simulink model "FFT4dSpace_1"  (R2021a)
settings: Solver=ode1  StartTime=0.0  StopTime=Inf  FixedStep=Ts  RelTol=1e-5
PostLoadFcn:
  | if any(exist('dsrtsu_mdlpostloadfcn', 'file') ~= 0), dsrtsu_mdlpostloadfcn('Execute', bdroot); end
InitFcn:
  | , if any(exist('rtifpga_mdlclblib', 'file') ~= 0), rtifpga_mdlclblib('Init', bdroot); end,
  | , if any(exist('dsmpb_private', 'file') ~= 0), dsmpb_private('dsmpb_mdlclblib', 'Init', bdroot); end,
values from neighbouring files (symbols this model uses):
  Ts_1kHz = 1e-3    (= 0.001)    [FFT4dSpace_1_i.m]
undefined symbols (not defined in the file or in its folder): CalibNormed, conv, mdlPara, PWMpara, Ro1_Be2, scaleHV, supplyPressure4VPPM
libraries: dsmpblib x46, tllib x2, dspxfrm3 x1, dspsigops x1
(part 1 of 2)
PreSaveFcn:
  | , if any(exist('dsmpb_private', 'file') ~= 0), dsmpb_private('dsmpb_mdlclblib', 'PreSave', bdroot); end,
CloseFcn:
  | , if any(exist('dsmpb_private', 'file') ~= 0), dsmpb_private('dsmpb_mdlclblib', 'Close', bdroot); end,
settings Model: TL_MAIN_DATA={'codeopt',{'globalbitfields',1,'cleancode',1},'logopt',{'globalloggingmode',4},'date',738813.6776019329,'advcodeopt',{'SupportSinglePrecisionLibraries';2}}  DS_PROJECTFILE=VEAE_Regler.dd  TLVersion=5.2.0.27  DSRTSU_INTERNAL_RTI_VER=580  DSRTSU_INTERNAL_RTI_TYPE=rti1202  RTICANMMDATA=struct('GeneralSetupData',struct('modelroot','C:\workspace\teachingSMC\FFT\dSpace\SCALEXIO','generalsettings',struct('filesettings',struct('destfolder',struct('Name','RTICANMM_FILES','Check',1),'buildfolder',struct('Name','.','Check',1),'AbsDestfolder',struct('Name','C:\workspace\teachingSMC\FFT\dSpace\SCALEXIO\RTICANMM_FILES'),'AbsBuildfolder',struct('Name','C:\workspace\teachingSMC\FFT\dSpace\SCALEXIO'))),'options',struct('addpaths',1,'rmpaths',1,'addtrcexclusion',true,'cannavigator',struct('checkmonitoring',0),'show_usrtrc',0,'use_usrtrc',0),'advanced',struct('options',ones(1,100)),'MPSetup',{{}},'RTI',struct('Type','DSRT','Ver','4.5','Date','02-May-2021'),'modelname','FFT4dSpace_1','block','FFT4dSpace_1'))  DSRTSU_INTERNAL_RTIFPGA=170  DSMPB_ID_DATA={'23691',struct('BlockId','e363dcf7-3c8b-40a0-94fa-9ca138f30a92','SignalIds',{{'8eaee084-b07d-4098-89ea-f14ffad18ffa'}}),'23692',struct('BlockId','33a1bf71-0d4c-4538-b9a6-2564a6bb3ed2','SignalIds',{{'7b532231-dc87-4623-a6bc-34b16234ae63'}}),'23693',struct('BlockId','80070c25-e06e-4fa7-bb77-63301d343f98','SignalIds',{{'1d35b1bf-c98b-4d88-ae94-1fc8c05d074d'}}),'23694',struct('BlockId','ad7704d0-4e59-4d7f-a1bb-c3e5207854ab','SignalIds',{{'30964f73-9c09-4fdc-bb51-0958be5a594d'}}),'23695',struct('BlockId','7aaee380-a7bb-4262-bf7a-0278c9ae6393','SignalIds',{{'cbf2b4e5-eba6-43e6-b587-c2127677f436'}}),'23696',struct('BlockId','36f2f2d5-5e42-4e25-9679-6cb3cb299ee5','SignalIds',{{'4b6b5e8b-c894-445c-bc7e-9990cb119b26'}}),'23697',struct('BlockId','71a2e424-6974-4253-bc43-95e389d7f603','SignalIds',{{'217da0a0-e3a9-4503-8c93-23feae479825'}}),'23698',struct('BlockId','8b7272b4-9be0-4b51-9ecb-302ecd5c3b3a','SignalIds',{{'4401bdaf-5b85-45f8-aa98-6959e1fe6847'}}),'23699',struct('BlockId','1db96408-7553-49ea-ae15-6e7e82f80655','SignalIds',{{'19da7aee-71cc-43f3-978b-66b6a099a4fa'}}),'23700',struct('BlockId','da4ac2f6-2b80-4d49-8dbf-3d2d4c3e429d','SignalIds',{{'0f867e66-a710-4dfd-aae0-36cd5f512122'}}),'23701',struct('BlockId','afd4257c-21a0-443f-8874-801e9e47d041','SignalIds',{{'ef4cd6d4-18a7-4dce-a9d8-4ae1aeb2dc70'}}),'23702',struct('BlockId','31438f08-e2ee-4bb4-abb9-b635e3636ed7','SignalIds',{{'7e1c8993-4ba1-482c-9dc1-fd8801ef3bb7'}}),'23722',struct('BlockId','bd682038-b3f1-451c-8889-2678fb1e0768','SignalIds',{{'8bc8299c-811b-4952-a633-8e6399a271bb','226ad07d-74a5-4348-9e16-0e760e13c5ea','fb77b335-58e6-40b8-9a39-c5d31b0115e1'}}),'23723',struct('BlockId','a9a2190b-8cc7-4831-ba2f-1a851ea58aef','SignalIds',{{'424d8948-39ab-4e70-baa5-0284423705d1','6157c886-271b-4e2c-9e64-a00fe997db60','bf2b604a-b232-4dca-951e-9f04b6190901'}}),'23724',struct('BlockId','4e0d0596-e847-41d4-ac4c-5549c7b68a70','SignalIds',{{'bcd34ae9-7391-4ec1-9116-0cf2ed083bb7','8dce8f9b-a3e1-43a5-9198-b0de8c72ab96','fd631e82-c4ba-420d-a832-f6f1a2e1fbf2'}}),'23725',struct('BlockId','b35cb07b-2765-4325-ba0e-4e1c0552a373','SignalIds',{{'bcc19acf-3645-4399-b2a6-a0b16bdb4434','a864334b-e486-47c0-b597-500b844d8df3','e9ee66d1-5c53-45d9-8a51-c60c45f2323a'}}),'23726',struct('BlockId','fc085d2d-a08d-447b-bb2c-55f41c3d2f58','SignalIds',{{'74f89104-11d1-44b2-9cce-5d5e36121983','58a323c5-8a29-4bfb-a24f-484cd4485a7a','a68058ee-dcad-46b1-af24-c0970f163968'}}),'23727',struct('BlockId','4f692a5d-2e07-4a4a-91aa-7aad3d22b323','SignalIds',{{'0b0ca5db-4351-48d9-aa89-15608aa96c34','c8c583e7-e575-4582-a023-d4cc5cccccc8','c457b778-0167-43a7-bc9f-1f9439149f83'}}),'23728',struct('BlockId','de7062cb-ec50-4fe6-ad2f-5964c9f43c03','SignalIds',{{'b0d0cdd9-a69b-4b2f-8686-152bd8c639ae','fd2f8604-b757-4c89-9a06-85e31da031f8','78e70a8d-34aa-48f6-9e91-9b7357999e14'}}),'23729',struct('BlockId','ee26962f-6483-47a5-9ae3-bdae23d41a82','SignalIds',{{'841699f9-1868-4e31-8b05-04831ea46d12','ef483acf-acac-49e3-bcf2-d459fa5b67e5','9a543403-5e94-4c76-83eb-20d980c5c198'}}),'23808',struct('BlockId','3618f7d3-770c-4d0b-a6f8-f57eef4aa707','SignalIds',{{'f887e2de-d35b-484c-8735-c498302bedaf'}}),'23809',struct('BlockId','d046d79b-4541-46bc-b50b-cbb132c517dd','SignalIds',{{'4adf8844-b3d9-48ac-afb0-aa431ebf3cfd'}}),'23810',struct('BlockId','9e33dab8-7c1e-4c10-8bac-9db27495f098','SignalIds',{{'c391cbb6-710b-41c5-a922-c0778a6fd7eb'}}),'23811',struct('BlockId','5047cf61-f79e-4571-babd-b46f8c31fe6f','SignalIds',{{'b6f989d1-85e3-4670-8a88-d8f123ece4d9'}}),'23812',struct('BlockId','84123028-2810-4ad1-975f-d307fc0b89eb','SignalIds',{{'9b0a0619-6ba6-4cbc-bb56-9b04bf7ffca0'}}),'23813',struct('BlockId','73b8bc57-ed34-4fde-ac01-a1e2ae6f212d','SignalIds',{{'f1bd759e-faf7-4478-8f9b-df97eda93df6'}}),'23814',struct('BlockId','02467e4c-1d3f-43c2-a575-9120e99575ea','SignalIds',{{'706fb417-39a5-419f-88e7-3d1a44326906'}}),'23815',struct('BlockId','30576d33-2aac-42bf-a78c-87ccc3cd6c01','SignalIds',{{'15c12989-3365-4ed1-9956-32a73db71a4d'}}),'23816',struct('BlockId','241ebb44-37d7-4bd2-a90d-0ea04f5a5d13','SignalIds',{{'f7f409fd-82fb-420b-ae76-eae684d90ce8'}}),'23817',struct('BlockId','fe42de6e-e6cd-4958-b6bb-718debe361a9','SignalIds',{{'2237635b-b2b4-4c94-86bb-2af412bd5cb8'}}),'23818',struct('BlockId','ea51ba60-b36a-4b1b-a248-4b35ae3fbf02','SignalIds',{{'80906cf2-aa07-496c-ab63-8acfe7b88759'}}),'23819',struct('BlockId','5e50a903-b4cf-479a-bba9-3e862b588a7a','SignalIds',{{'f80be48e-04e0-4bbc-94b1-e70b4d66f511'}}),'23820',struct('BlockId','7e573d54-38f9-41cf-a1ec-944dbb580650','SignalIds',{{'18737848-b3cc-470c-bff3-c14923aeca9b'}}),'23821',struct('BlockId','b40408dc-1d09-4b5e-b237-16e8872f357c','SignalIds',{{'381221ba-92f7-452a-8919-a8dd194524f7'}}),'23822',struct('BlockId','ac12e463-1157-45c4-a832-8a5484798087','SignalIds',{{'a20ec9ef-3c4b-4516-80e6-aea48d0d4a5c'}}),'23823',struct('BlockId','12f2115a-32be-4530-8d50-170bd71868ca','SignalIds',{{'394d649a-f46e-4805-83d9-d6cef483b7cd'}}),'23824',struct('BlockId','4e6ca114-81cb-481c-a0bb-b1573ff8e678','SignalIds',{{'da560366-0282-4fe5-94a0-da07a126ccc6'}}),'23825',struct('BlockId','6b18697c-40d5-402c-b9f7-e49b1f7cf619','SignalIds',{{'e3ede30a-e584-4b21-8fd4-4e675ebea708'}}),'23826',struct('BlockId','858f3f7c-a976-4e60-9a36-a5ba33175241','SignalIds',{{'e0824d91-0663-4ea2-af54-0f949cc3e418'}}),'23827',struct('BlockId','42c052ba-50d6-4985-9edf-50fac3901a3e','SignalIds',{{'2b1dcab9-ca84-4da1-a49d-55d11d9371e8'}}),'24118',struct('BlockId','47a249fb-d4e0-4e70-a5f5-36e301043995','SignalIds',{{'13cad4c5-6086-4e10-9ce6-5cdb82307704'}}),'24119',struct('BlockId','46dd8d37-e2a1-439f-89fc-ea00411d4ca3','SignalIds',{{'bbc1bd72-d794-442b-b6e2-735ad3ac33cb'}}),'24120',struct('BlockId','2aa52a3b-223d-4687-aa02-e1a44ea5c063','SignalIds',{{'bbf5d31c-0351-4836-994a-4c8856759900','550d0838-0baa-4757-a0e1-c46c9a3232a3'}}),'24121',struct('BlockId','995ad4dd-aaa8-465e-98cc-2dc6b2417123','SignalIds',{{'c825e840-241a-4b6f-bf2c-380bbaca74e6','5c01308f-615e-4599-acb8-22a35f81ada1'}}),'24122',struct('BlockId','885bc184-7968-4b50-898b-f403f006dcca','SignalIds',{{'6d9af1df-5ae3-49ad-ae84-01a7f8537bb7'}}),'25475',struct('BlockId','44a8e465-c9c5-409d-b2e8-7dd00d563f6d','SignalIds',{{'90fb2f1b-7fef-4790-ba3c-b5681fb51816','785fae22-0f32-4539-84e4-b96917a39273','b1ae88c2-cc42-4767-b4a8-823d65a01f97','176642e3-a060-49ad-bb31-43627c94ec8c','44d0cc4c-38bd-49d8-a6ec-c2148defedc4','7e07ee8a-8bd1-4ee4-aff1-5057cefc46ce'}})}  Creator=mibr  LastModifiedBy=nitr
settings SolverCC: AlgebraicLoopSolver=TrustRegion
settings DataIOCC: SaveFormat=Array  SaveOutput=off  DSMLogging=off  SaveTime=off  ReturnWorkspaceOutputs=off
settings OptimizationCC: BlockReduction=off  ConditionallyExecuteInputs=off  OptimizeBlockIOStorage=off  BufferReuse=off  GlobalBufferReuse=off  ExpressionFolding=off  LocalBlockOutputs=off  OptimizeDataStoreBuffers=off  BusAssignmentInplaceUpdate=off
settings DebuggingCC: SolverPrmCheckMsg=warning  TasksWithSamePriorityMsg=none  ParameterPrecisionLossMsg=none  UniqueDataStoreMsg=error  BusObjectLabelMismatch=error  StrictBusMsg=ErrorOnBusTreatedAsVector  NonBusSignalsTreatedAsBus=error  SFUnexpectedBacktrackingDiag=warning  SFNoUnconditionalDefaultTransitionDiag=warning  SFExecutionAtInitializationDiag=none  SFMachineParentedDataDiag=warning  ArithmeticOperatorsInVariantConditions=warning
settings HardwareCC: ProdBitPerPointer=32  ProdBitPerSizeT=32  ProdBitPerPtrDiffT=32  ProdLargestAtomicInteger=Integer  ProdWordSize=32  ProdLongLongMode=on  ProdHWDeviceType=Custom Processor->Custom  TargetIntDivRoundTo=Zero  TargetEndianess=BigEndian  TargetHWDeviceType=Custom Processor->Custom
settings ModelReferenceCC: EnableParallelModelReferenceBuilds=on
settings SFSimCC: MATLABDynamicMemAlloc=off  CustomCodeUndefinedFunction=UseInterfaceOnly
settings RTWCC: Description=dSPACE Run-Time Target (for VEOS on Windows and ConfigurationDesk)  SystemTargetFile=dsrt.tlc  GenCodeOnly=on  MakeCommand=make_dsrt  TemplateMakefile=dsrt_default_tmf  RTWVerbose=off
settings CodeAppCC: StateflowObjectComments=on
settings STFCustomTargetCC: ParMdlRefBuildCompliant=on  GRTInterface=off  UseToolchainInfoCompliant=off  SystemTargetFile=dsrt.tlc
settings GRTTargetCC: TargetLangStandard=C89/C90 (ANSI)  CompOptLevelCompliant=off  ConcurrentExecutionCompliant=off  CombineOutputUpdateFcns=off  MatFileLogging=off  CPPClassGenCompliant=off  UseToolchainInfoCompliant=off

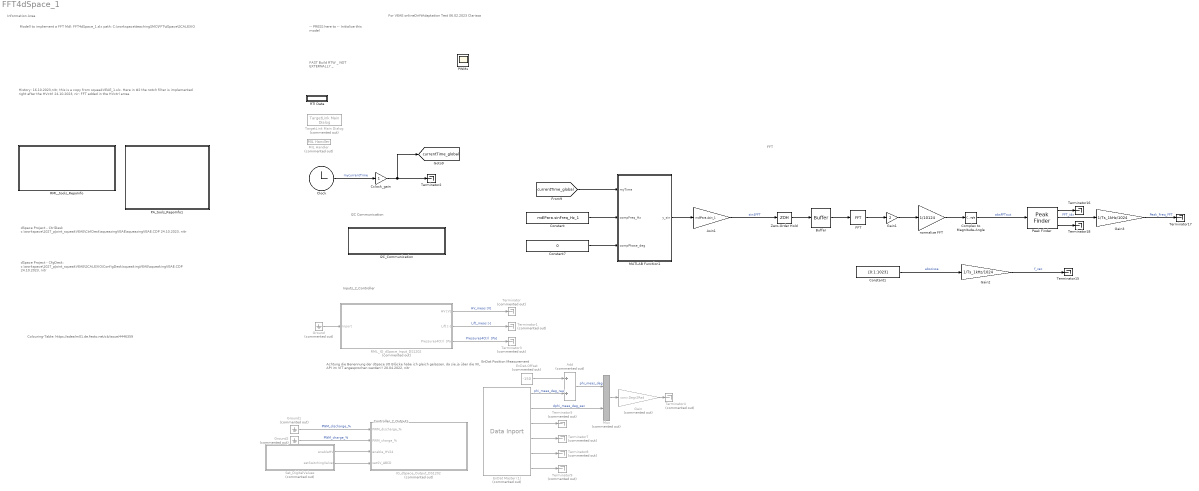
== system FFT4dSpace_1 ==
  note: Colouring-Table:
      | https://adealm01.de.festo.net/cb/issue/4446359
  note: EnDat Position Measurement
  note: For VEAE onlineDriftAdaptation Test
      | 06.02.2023
      |
      | Clarissa
  note: Achtung die Benennung der dSpace I/O Blöcke
      | habe ich gleich gelassen, da sie ja über die XIL API im VIT angesprochen werden!!
      |
      | 20.04.2022, nitr
  note: FAST Build RTW
      | _ NOT EXTERNALLY _
  note: Information Area
  note: dSpace Project - CtrlDesk
      | c:\workspace\1027_pJoint_squeakVEAE\CtrlDesk\squeazingVEAE\squeazingVEAE.CDP
      | 24.10.2023, nitr
  note: History:
      |
      | 16.10.2023,nitr, this is a copy from squeakVEAE_1.slx. Here in #2 the notch filter is implemented
      | right after the HVctrl
      | 24.10.2023, nir: FFT added in the HVctrl arrea
  note: Controller_2_Outputs
  note: -- PRESS here to --
      | Initialize this model
  note: Modell to implement a FFT
      |
      | Mdl: FFT4dSpace_1.slx
      | path: C:\workspace\teachingSMC\FFT\dSpace\SCALEXIO
  note: Inputs_2_Controller
  note: dSpace Project - CfgDesk:
      |
      | c:\workspace\1027_pJoint_squeakVEAE\SCALEXIO\ConfigDesk\squeakingVEAE\squeakingVEAE.CDP
      | 24.10.2023, nitr
  note: I2C Communication
  note: FFT
  Add : Sum  Commented=on
  Asin1 : Gain  Gain=mdlPara.Asin_1
  Buffer : Buffer  N=1024  OutputFrames=off
  Cclock_gain : Gain
  Clock : Clock
  Complex to Magnitude-Angle : ComplexToMagnitudeAngle  Output=Magnitude
  Constant : Constant  Value=mdlPara.sinFreq_Hz_1
  Constant1 : Constant  Value=[0:1:1023]
  Constant7 : Constant  Value=0
  EnDat Master (1) : dsmpblib/Data Inport  Priority=10000  Commented=on
      settings: SourceProductName=dSPACE Model Interface Blockset
  EnDat-Offset : Constant  Commented=on  Value=-150
  FFT : dspxfrm3/FFT  FFTImplementation=Auto  CompMethod=Table lookup  TableOpt=NEW  TableOptActive=Speed  BitRevOrder=off  Normalize=off  InheritFFTLength=on  FFTLength=64  WrapInput=on  roundingMode=Floor  overflowMode=off  firstCoeffDataTypeStr=Inherit: Same word length as input  firstCoeffLastDataTypeStr=Inherit: Same word length as input  outputMin=[]  outputMax=[]
  Gain : Gain  Commented=on  Gain=conv.Degr2Rad
  Gain1 : Gain  Gain=2
  Gain2 : Gain  Gain=1/Ts_1kHz/1024
  Gain3 : Gain  Gain=1/Ts_1kHz/1024
  Ground : Ground  Commented=on
  Ground1 : Ground  Commented=on
  Ground2 : Ground  Commented=on
  I2C_Communication : Subsystem
  IO_dSpace_Output_DS1202 : Subsystem  Tag=PA_IO_dSpace_Output_DS1513  Commented=on  mask(PA_dSpace_Output_DS1513){}
      mask help:
      | This block contains all outputsignals from dSpace RTI 1401. This Block
      | is a template. Before using in the block break the link to the library!
      | After breaking it is possible to connect the input with the block.
      |
      | It contains the signals:
      |
      | PWM_OUT1 ... PWM_OUT4
      | DIG_OUT1 ... DIG_OUT3
      | DAC1 ... DAC4
      mask Help: eval(['run(strcat(''',getenv('pasl_simulink'),''',''\documentation\tools\HelpForPaslElements.m''))']);
      mask Display: image('dSpaceInOut_rti1202_out.png')
  MATLAB Function1 : MATLAB Function  TreatAsAtomicUnit=on
  MIL Handler : tllib/MIL Handler  Commented=on  data={'date',738813.67760843749}
      settings: SourceProductName=dSPACE TargetLink common blockset
  Mux : Mux  Commented=on  Inputs=2
  PA_tools_RepoInfo1 : Subsystem  Tag=RevTagSubSys  mask(cover){}
      mask help: mask for library reasons
      settings: OpenFcn=PA_setRepoInfoBlock()
      mask Help: eval(['run(strcat(''',getenv('pasl_simulink'),''',''\documentation\tools\HelpForPaslElements.m''))']);
      mask Display: text(.05,.95,'Project:\n   Rev#:  8\n   RevID: 7424ff1b57da\n   date:  Mon, 23 Oct 2023 16:39:53 +0200\n   branch:  master\n\nPASL:\n   Rev#:  708\n   RevID: e154c95b446a\n   date:  Thu, 19 May 2022 11:39:18 +0200\n   branch:  master\n\nPATL:\n   Rev#:  144\n   RevID: 47544a47bed1\n   date:  Thu, 28 Apr 2022 22:19:34 +0200\n   branch:  master\n\nPADL:\n   Rev#:  UNKNOWN\n   RevID: UNKNOWN\n   date:  UNKNOWN\n   branch:  UNKNOWN\n\n','hor','left','ver','top')
  Peak Finder : dspsigops/Peak Finder  polarity=Maxima  indexBase=Zero  outputIdx=on  outputVal=on  maxPeaks=3  NoiseDistinguish=on  thresh=mdlPara.thres4peak  roundingMode=Floor  overflowMode=off
      settings: SourceProductBaseCode=DS  allowOverrides=off
  RML_IO_dSpace_Input_DS1202 : Subsystem  Commented=on
      mask Display: image('dSpaceInOut_rti1202_in.png')
  RML_tools_RepoInfo : Subsystem  Tag=rmlRevTagSubSys  mask(cover){}
      mask help: mask for library reasons
      settings: OpenFcn=rmlSetRepoInfoBlock()
      mask Help: eval(['run(strcat(''',getenv('rml_root'),'\documentation\tools\rmlHelpForRmlElements.m''))'])
      mask Display: text(.05,.95,'Project:\n   Rev#:  8\n   RevID: 7424ff1b57da\n   date:  Mon, 23 Oct 2023 16:39:53 +0200\n   branch:  master\n\nRML:\n   Rev#:  736\n   RevID: 95e677d319d7\n   date:  Fri, 24 Feb 2023 13:39:56 +0100\n   branch:  develop\n\n','hor','left','ver','top')
  RTI Data : Subsystem  Tag=struct('RTIDataServer',struct('RTIDataServerVs','2','RTIModelDescription','struct(''main'',''FFT4dSpace_1'',''sub'',''FFT4dSpace_1'',''isMp'',0)'))  LoadFcn="if exist('rtidc'), try,  rtidc('DataHostBlockClbLoad', gcbh); catch, disp(['Warning: ''LoadFcn'' for RTI Data block failed: ' lasterr]); end, end,"  mask(RTI_DATA_HOST){}
      mask help:
      | RTI Data Block.
      | This block is used by RTI to store internal model-dependent data.
      | Please keep this block on the root level of the model. Deleting this block will result in data loss.
      |
      | NEVER DELETE OR COPY THIS BLOCK!
      settings: CopyFcn="if exist('rtidc'), try,  rtidc('DataHostBlockClbCopy', gcbh); catch, disp(['Warning: ''CopyFcn'' for RTI Data block failed: ' lasterr]); end, end,"  DeleteFcn="if exist('rtidc'), try,  rtidc('DataHostBlockClbDelete', gcbh); catch, disp(['Warning: ''DeleteFcn'' for RTI Data block failed: ' lasterr]); end, end,"  ModelCloseFcn="if exist('rtidc'), try,  rtidc('DataHostBlockClbModelClose', gcbh); catch, disp(['Warning: ''ModelCloseFcn'' for RTI Data block failed: ' lasterr]); end, end,"  PreSaveFcn="if exist('rtidc'), try,  rtidc('DataHostBlockClbPreSave', gcbh); catch, disp(['Warning: ''PreSaveFcn'' for RTI Data block failed: ' lasterr]); end, end,"  PostSaveFcn="if exist('rtidc'), try,  rtidc('DataHostBlockClbPostSave', gcbh); catch, disp(['Warning: ''PostSaveFcn'' for RTI Data block failed: ' lasterr]); end, end,"  NameChangeFcn="if exist('rtidc'), try,  rtidc('DataHostBlockClbNameChange', gcbh); catch, disp(['Warning: ''NameChangeFcn'' for RTI Data block failed: ' lasterr]); end, end,"
      mask Help:
      | RTI Data Block.
      | This block is used by RTI to store internal model-dependent data.
      | Please keep this block on the root level of the model. Deleting this block will result in data loss.
      | 
      | NEVER DELETE OR COPY THIS BLOCK!
      mask Display:
      | text(0.5, 0.5, 'RTI Data', 'HorizontalAlignment', 'center');
      | plot([1 0]);
  Set_DigitalValues : Subsystem  Commented=on
  TargetLink Main Dialog : tllib/TargetLink Main Dialog  Commented=on  data=[]
      settings: SourceProductName=dSPACE TargetLink common blockset
  Terminator{,1,3..5,7..9} (8 alike) : Terminator  Commented=on
  Terminator{2,15..18} (5 alike) : Terminator
  Zero-Order Hold : ZeroOrderHold  SampleTime=Ts_1kHz
  normalize FFT : Gain  Gain=1/10124
  PWMs : Scope
  tag scope: currentTime_global=global
  wires:
  Ground2/1 -> IO_dSpace_Output_DS1202/2(PWM_charge_%)  "PWM_charge_%"
  RML_IO_dSpace_Input_DS1202/1(HV [V]) -> Terminator/1  "HV_meas [V]"
  RML_IO_dSpace_Input_DS1202/2(Lift [-]) -> Terminator1/1  "Lift_meas [-]"
  RML_IO_dSpace_Input_DS1202/3(Pressures4Ctrl  [Pa]) -> Terminator3/1  "Pressures4Ctrl  [Pa]"
  Ground1/1 -> IO_dSpace_Output_DS1202/1(PWM_discharge_%)  "PWM_discharge_%"
  Set_DigitalValues/1("enableHV ") -> IO_dSpace_Output_DS1202/3(enable_HV24)
  Set_DigitalValues/2(setSwitchingValves) -> IO_dSpace_Output_DS1202/4(setSV_ABCD)
  Clock/1 -> Cclock_gain/1  "mycurrentTime"
  Cclock_gain/1 -> [currentTime_global], Terminator2/1
  EnDat Master (1)/2 -> Mux/2  "dphi_meas_deg_sec"
  EnDat Master (1)/3 -> Terminator5/1
  EnDat Master (1)/4 -> Terminator7/1
  EnDat Master (1)/5 -> Terminator8/1
  EnDat Master (1)/6 -> Terminator9/1
  EnDat Master (1)/1 -> Add/2  "phi_meas_deg_raw"
  EnDat-Offset/1 -> Add/1
  Gain/1 -> Terminator4/1
  Mux/1 -> Gain/1
  Add/1 -> Mux/1  "phi_meas_deg"
  Ground/1 -> RML_IO_dSpace_Input_DS1202/1(Inport)
  Complex to Magnitude-Angle/1 -> Peak Finder/1  "absFFTout"
  Peak Finder/2 -> Gain3/1  "FFT_idx"
  Peak Finder/3 -> Terminator18/1
  FFT/1 -> Gain1/1
  normalize FFT/1 -> Complex to Magnitude-Angle/1
  Gain3/1 -> Terminator17/1  "Peak_Freq_FFT"
  Buffer/1 -> FFT/1
  Constant1/1 -> Gain2/1  "abscissa"
  Gain1/1 -> normalize FFT/1
  Gain2/1 -> Terminator15/1  "f_vec"
  Peak Finder/1 -> Terminator16/1
  Zero-Order Hold/1 -> Buffer/1
  Constant7/1 -> MATLAB Function1/3(compPhase_deg)
  Constant/1 -> MATLAB Function1/2(compFreq_Hz)
  [currentTime_global] -> MATLAB Function1/1(myTime)
  MATLAB Function1/1(y_sin) -> Asin1/1
  Asin1/1 -> Zero-Order Hold/1  "sin4FFT"

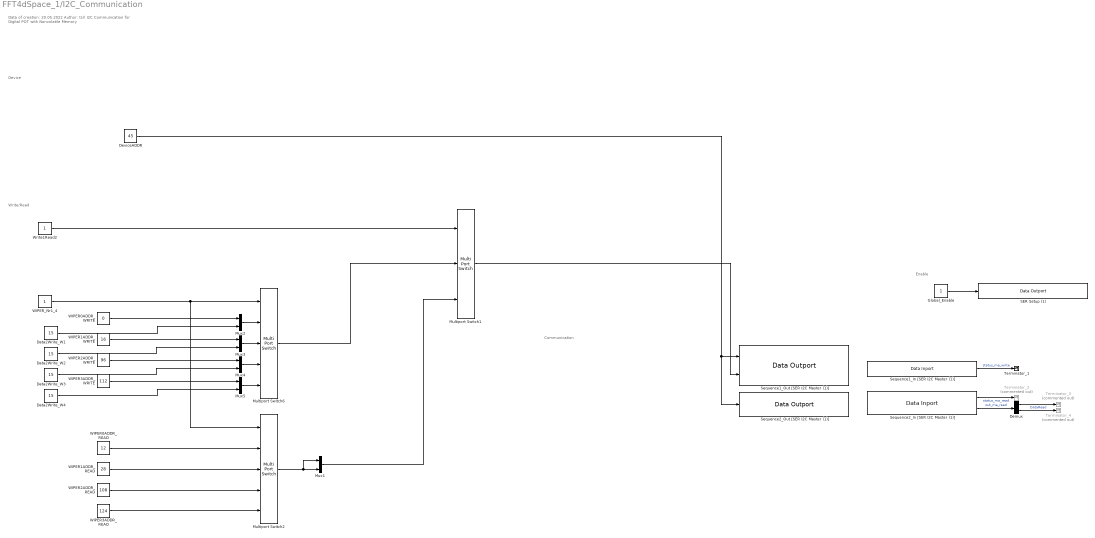
== system FFT4dSpace_1/I2C_Communication ==
  note: Data of creation: 20.05.2022
      | Author: tsrl
      |
      | I2C Communication for Digital POT with Nonvolatile Memory
  note: Enable
  note: Device
  note: Communication
  note: Write/Read
  Data2Write_W{1..4} (4 alike) : Constant  Value=15
  Demux : Demux  Outputs=2
  DeviceADDR : Constant  Value=45
  Global_Enable : Constant
  Multiport Switch1 : MultiPortSwitch  Inputs=2
  Multiport Switch2 : MultiPortSwitch  Inputs=4
  Multiport Switch6 : MultiPortSwitch  Inputs=4
  Mux{1..5} (5 alike) : Mux  Inputs=2
  SER Setup (1) : dsmpblib/Data Outport  Priority=-10000
      settings: SourceProductName=dSPACE Model Interface Blockset
  Sequence1_In [SER I2C Master (1)] : dsmpblib/Data Inport  Priority=10000
      settings: SourceProductName=dSPACE Model Interface Blockset
  Sequence1_Out [SER I2C Master (1)] : dsmpblib/Data Outport  Priority=-10000
      settings: SourceProductName=dSPACE Model Interface Blockset
  Sequence2_In [SER I2C Master (1)] : dsmpblib/Data Inport  Priority=10000
      settings: SourceProductName=dSPACE Model Interface Blockset
  Sequence2_Out [SER I2C Master (1)] : dsmpblib/Data Outport  Priority=-10000
      settings: SourceProductName=dSPACE Model Interface Blockset
  Terminator_1 : Terminator
  Terminator_2 : Terminator  Commented=on
  Terminator_3 : Terminator  Commented=on
  Terminator_4 : Terminator  Commented=on
  WIPER0ADDR_READ : Constant  Value=12
  WIPER0ADDR_WRITE : Constant  Value=0
  WIPER1ADDR_READ : Constant  Value=28
  WIPER1ADDR_WRITE : Constant  Value=16
  WIPER2ADDR_READ : Constant  Value=108
  WIPER2ADDR_WRITE : Constant  Value=96
  WIPER3ADDR_READ : Constant  Value=124
  WIPER3ADDR_WRITE : Constant  Value=112
  WIPER_Nr1_4 : Constant
  Write1Read2 : Constant
  wires:
  WIPER_Nr1_4/1 -> Multiport Switch2/1, Multiport Switch6/1
  Global_Enable/1 -> SER Setup (1)/1
  Sequence1_In [SER I2C Master (1)]/1 -> Terminator_1/1  "status_ma_write"
  WIPER3ADDR_READ/1 -> Multiport Switch2/5
  WIPER1ADDR_READ/1 -> Multiport Switch2/3
  Sequence2_In [SER I2C Master (1)]/1 -> Terminator_2/1  "status_ma_read"
  Multiport Switch2/1 -> Mux1/1, Mux1/2
  Mux1/1 -> Multiport Switch1/3
  WIPER2ADDR_READ/1 -> Multiport Switch2/4
  Write1Read2/1 -> Multiport Switch1/1
  WIPER0ADDR_READ/1 -> Multiport Switch2/2
  Demux/2 -> Terminator_4/1  "DataRead"
  DeviceADDR/1 -> Sequence2_Out [SER I2C Master (1)]/1, Sequence1_Out [SER I2C Master (1)]/1
  Multiport Switch1/1 -> Sequence1_Out [SER I2C Master (1)]/2
  Sequence2_In [SER I2C Master (1)]/2 -> Demux/1  "out_ma_read"
  Demux/1 -> Terminator_3/1
  Multiport Switch6/1 -> Multiport Switch1/2
  WIPER0ADDR_WRITE/1 -> Mux2/1
  Data2Write_W1/1 -> Mux2/2
  WIPER1ADDR_WRITE/1 -> Mux3/1
  WIPER2ADDR_WRITE/1 -> Mux4/1
  WIPER3ADDR_WRITE/1 -> Mux5/1
  Data2Write_W2/1 -> Mux3/2
  Data2Write_W3/1 -> Mux4/2
  Data2Write_W4/1 -> Mux5/2
  Mux2/1 -> Multiport Switch6/2
  Mux3/1 -> Multiport Switch6/3
  Mux4/1 -> Multiport Switch6/4
  Mux5/1 -> Multiport Switch6/5

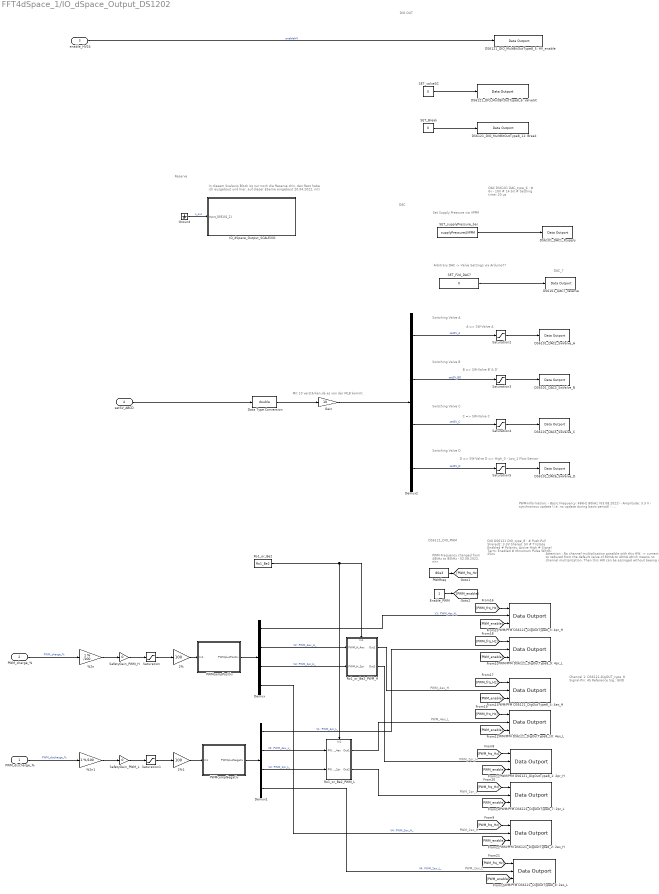
== system FFT4dSpace_1/IO_dSpace_Output_DS1202 ==
  note: A => SW-Valve A
  note: Reserve
  note: PWM Frequency changed from 48kHz to 80kHz - 02.08.2022, nitr
  note: In diesem Scalexio Block ist nur noch die Reserve drin,
      | den Rest habe ich ausgebaut und hier, auf dieser Eberne eingebaut
      | 20.04.2022, nitr
  note: Mit 10 verstärken,da es von der MLB kommt.
  note: Arbitrary DAC -> Valve Settings via Arduino??
  note: Set Supply Pressure via VPPM
  note: DAC
  note: DIG OUT
  note: PWM_4ex_H
  note: PWM_4ex_L
  note: PWM_2ex_H
  note: PWM_2pr_L
  note: PWM_2pr_H
  note: PWM_2ex_L
  note: DAC_7
  note: Switching Valve A
  note: Switching Valve B
  note: Switching Valve C
  note: Switching Valve D
  note: DAC DS6101 DAC_type_6 :
      | # 0v - 10V
      | # 14 bit
      | # Settling time: 20 µs
  note: DIO DS6121 DIO_type_8 :
      | # Push-Pull
      | Shared2: 3.3V
      | Shared: 5V
      | # Tristate Enabled
      | # Polarity: Active High
      | # Signal Term: Enabled
      |
      | # Minumum Pulse Witdh: 25ns
  note: Channel 1: DS6121-DigOUT_type_8
      | Signal-Pin: 45
      | Reference Sig.: GND
  note: PWM-Information:
      | - Basic Frequency: 48kHz 80kHz (03.08.2022)
      | - Amplitude: 3.3 V
      | - synchronous update (i.e. no update during basis period)
      | - ....
  note: DS6121_DIO_PWM
  note: Attention :
      | No channel multiplication possible with this HW,
      | -> current has to reduced from the default value of 80mA to 40mA
      | which means no channel multiplication. Then this HW can be assinged
      | without beeing red :)
  note: B => SW-Valve B' & D'
  note: C => SW-Valve C
  note: D => SW-Valve D => High_0 - Low_1 Flow Sensor
  PWM_discharge_% : Inport
  PWM_charge_% : Inport  Port=2
  enable_HV24 : Inport  Port=3
  setSV_ABCD : Inport  Port=4
  %2n : Gain  Gain=1 % /100
  %2n1 : Gain  Gain=1 %/100
  2% : Gain  Gain=100
  2%1 : Gain  Gain=100
  DS6101_DAC1_Psupply : dsmpblib/Data Outport  Priority=-10000
      settings: SourceProductName=dSPACE Model Interface Blockset
  DS6101_DAC2_SwValve_A : dsmpblib/Data Outport  Priority=-10000
      settings: SourceProductName=dSPACE Model Interface Blockset
  DS6101_DAC3_SwValve_B : dsmpblib/Data Outport  Priority=-10000
      settings: SourceProductName=dSPACE Model Interface Blockset
  DS6101_DAC5_SwValve_C : dsmpblib/Data Outport  Priority=-10000
      settings: SourceProductName=dSPACE Model Interface Blockset
  DS6101_DAC6_SwValve_D : dsmpblib/Data Outport  Priority=-10000
      settings: SourceProductName=dSPACE Model Interface Blockset
  DS6101_DAC7_reserve : dsmpblib/Data Outport  Priority=-10000
      settings: SourceProductName=dSPACE Model Interface Blockset
  DS6121_DIO_MultBitOutType8_11: Break : dsmpblib/Data Outport  Priority=-10000
      settings: SourceProductName=dSPACE Model Interface Blockset
  DS6121_DIO_MultBitOutType8_5: HV_enable : dsmpblib/Data Outport  Priority=-10000
      settings: SourceProductName=dSPACE Model Interface Blockset
  DS6121_DIO_MultBitOutType8_6: valveSC : dsmpblib/Data Outport  Priority=-10000
      settings: SourceProductName=dSPACE Model Interface Blockset
  Data Type Conversion : DataTypeConversion  OutDataTypeStr=double
  Demux : Demux
  Demux1 : Demux
  Demux2 : Demux
  Enable_PWM : Constant
  Gain : Gain  Gain=10
  Ground : Ground
  IO_dSpace_Output_SCALEXIO : Subsystem
      mask Display: image('dSpace_output.png')
  PWM/PFM DS6121_DigOutType8_10: 4ex_L : dsmpblib/Data Outport  Priority=-10000
      settings: SourceProductName=dSPACE Model Interface Blockset
  PWM/PFM DS6121_DigOutType8_1: 2pr_H : dsmpblib/Data Outport  Priority=-10000
      settings: SourceProductName=dSPACE Model Interface Blockset
  PWM/PFM DS6121_DigOutType8_2: 2ex_H : dsmpblib/Data Outport  Priority=-10000
      settings: SourceProductName=dSPACE Model Interface Blockset
  PWM/PFM DS6121_DigOutType8_3: 4pr_H : dsmpblib/Data Outport  Priority=-10000
      settings: SourceProductName=dSPACE Model Interface Blockset
  PWM/PFM DS6121_DigOutType8_4: 4ex_H : dsmpblib/Data Outport  Priority=-10000
      settings: SourceProductName=dSPACE Model Interface Blockset
  PWM/PFM DS6121_DigOutType8_7: 2pr_L : dsmpblib/Data Outport  Priority=-10000
      settings: SourceProductName=dSPACE Model Interface Blockset
  PWM/PFM DS6121_DigOutType8_8: 2ex_L : dsmpblib/Data Outport  Priority=-10000
      settings: SourceProductName=dSPACE Model Interface Blockset
  "PWM/PFM DS6121_DigOutType8_9: 4pr_L " : dsmpblib/Data Outport  Priority=-10000
      settings: SourceProductName=dSPACE Model Interface Blockset
  PWMcompNegativ : Subsystem
  PWMcompPositiv : Subsystem
  PWMfreq : Constant  Value=80e3
  Ro1_or_Be2 : Constant  Value=Ro1_Be2
  Ro1_or_Be2_PWM_H : Subsystem
      settings: PortSchema="{\"entries\":[{\"content\":{\"sides\":[{\"content\":{\"connectorIds\":[\"In1\",\"In2\"]},\"type\":\"ConnectorPlacement.EquallySpacedRectSide\",\"uuid\":\"33d120dc-88df-47e4-aceb-bf4939cbf745\"},{\"content\":{\"connectorIds\":[\"Out1\",\"Out2\"],\"side\":\"RIGHT\"},\"type\":\"ConnectorPlacement.EquallySpacedRectSide\",\"uuid\":\"b0000f29-fcf7-4c5a-a30f-88f0f10b005c\"},{\"content\":{\"connectorIds\":[\"In3\"],\"side\":\"TOP\"},\"type\":\"ConnectorPlacement.EquallySpacedRectSide\",\"uuid\":\"c9d41a43-30b6-47f1-b750-b85244b1e24d\"}]},\"type\":\"ConnectorPlacement.EquallySpacedConnector\",\"uuid\":\"b94f8a7b-aafd-4e61-9282-ebe0205f7a66\"}],\"packageUris\":[\"http://schema.mathworks.com/mf0/Connector/R2020b\"],\"version\":\"1.0\"}"
  Ro1_or_Be2_PWM_L : Subsystem
      settings: PortSchema="{\"entries\":[{\"content\":{\"sides\":[{\"content\":{\"connectorIds\":[\"In1\",\"In2\"]},\"type\":\"ConnectorPlacement.EquallySpacedRectSide\",\"uuid\":\"33d120dc-88df-47e4-aceb-bf4939cbf745\"},{\"content\":{\"connectorIds\":[\"Out1\",\"Out2\"],\"side\":\"RIGHT\"},\"type\":\"ConnectorPlacement.EquallySpacedRectSide\",\"uuid\":\"b0000f29-fcf7-4c5a-a30f-88f0f10b005c\"},{\"content\":{\"connectorIds\":[\"In3\"],\"side\":\"TOP\"},\"type\":\"ConnectorPlacement.EquallySpacedRectSide\",\"uuid\":\"c9d41a43-30b6-47f1-b750-b85244b1e24d\"}]},\"type\":\"ConnectorPlacement.EquallySpacedConnector\",\"uuid\":\"b94f8a7b-aafd-4e61-9282-ebe0205f7a66\"}],\"packageUris\":[\"http://schema.mathworks.com/mf0/Connector/R2020b\"],\"version\":\"1.0\"}"
  SET_Break : Constant  Value=0  OutDataTypeStr=boolean
  SET_F2d_DAC7 : Constant  Value=0
  SET_supplyPressure_bar : Constant  Value=supplyPressure4VPPM
  SET_valveSC : Constant  Value=0  OutDataTypeStr=boolean
  SafetyGain_PWM_H : Gain  Gain=0
  SafetyGain_PWM_L : Gain  Gain=0
  Saturation : Saturate  UpperLimit=1  LowerLimit=0
  Saturation1 : Saturate  UpperLimit=1  LowerLimit=0
  Saturation{2..5} (4 alike) : Saturate  UpperLimit=10  LowerLimit=0
  wires:
  Demux2/4 -> Saturation5/1  "setSV_D"
  Demux2/3 -> Saturation4/1  "setSV_C"
  Demux2/2 -> Saturation3/1  "setSV_BD"
  Demux2/1 -> Saturation2/1  "setSV_A"
  SET_supplyPressure_bar/1 -> DS6101_DAC1_Psupply/1
  PWM_charge_%/1 -> %2n/1  "PWM_charge_%"
  PWM_discharge_%/1 -> %2n1/1  "PWM_discharge_%"
  %2n/1 -> SafetyGain_PWM_H/1
  %2n1/1 -> SafetyGain_PWM_L/1
  Demux/2 -> Ro1_or_Be2_PWM_H/1(PWM_H_4ex)  "V2: PWM_4ex_H_"
  Demux/1 -> PWM/PFM DS6121_DigOutType8_3: 4pr_H/2  "V1: PWM_4pr_H_"
  Demux/3 -> Ro1_or_Be2_PWM_H/2(PWM_H_2pr)  "V3: PWM_2pr_H_"
  Demux/4 -> PWM/PFM DS6121_DigOutType8_2: 2ex_H/2  "V4: PWM_2ex_H_"
  setSV_ABCD/1 -> Data Type Conversion/1
  Demux1/4 -> PWM/PFM DS6121_DigOutType8_8: 2ex_L/2  "V4: PWM_2ex_L_"
  Demux1/1 -> "PWM/PFM DS6121_DigOutType8_9: 4pr_L "/2  "V1: PWM_4pr_L_"
  Demux1/2 -> Ro1_or_Be2_PWM_L/1(PWM_L_4ex)  "V2: PWM_4ex_L_"
  SafetyGain_PWM_H/1 -> Saturation/1
  Saturation/1 -> 2%/1
  SafetyGain_PWM_L/1 -> Saturation1/1
  Saturation1/1 -> 2%1/1
  enable_HV24/1 -> DS6121_DIO_MultBitOutType8_5: HV_enable/1  "enableHV"
  SET_F2d_DAC7/1 -> DS6101_DAC7_reserve/1
  Saturation2/1 -> DS6101_DAC2_SwValve_A/1
  Saturation3/1 -> DS6101_DAC3_SwValve_B/1
  Saturation4/1 -> DS6101_DAC5_SwValve_C/1
  Saturation5/1 -> DS6101_DAC6_SwValve_D/1
  Data Type Conversion/1 -> Gain/1
  Demux1/3 -> Ro1_or_Be2_PWM_L/2(PWM_L_2pr)  "V3: PWM_2pr_L_"
  Ro1_or_Be2/1 -> Ro1_or_Be2_PWM_L/3(In1), Ro1_or_Be2_PWM_H/3(In1)
  Ground/1 -> IO_dSpace_Output_SCALEXIO/1(Input_DS6101_21)  "s_out"
  Gain/1 -> Demux2/1
  [PWM_enable] -> PWM/PFM DS6121_DigOutType8_4: 4ex_H/3
  [PWM_enable] -> PWM/PFM DS6121_DigOutType8_1: 2pr_H/3
  Enable_PWM/1 -> [PWM_enable]
  [PWM_enable] -> PWM/PFM DS6121_DigOutType8_3: 4pr_H/3
  [PWM_frq_Hz] -> PWM/PFM DS6121_DigOutType8_7: 2pr_L/1
  [PWM_enable] -> "PWM/PFM DS6121_DigOutType8_9: 4pr_L "/3
  [PWM_frq_Hz] -> PWM/PFM DS6121_DigOutType8_4: 4ex_H/1
  [PWM_frq_Hz] -> PWM/PFM DS6121_DigOutType8_10: 4ex_L/1
  [PWM_frq_Hz] -> "PWM/PFM DS6121_DigOutType8_9: 4pr_L "/1
  Ro1_or_Be2_PWM_L/2(Out2) -> PWM/PFM DS6121_DigOutType8_7: 2pr_L/2
  [PWM_frq_Hz] -> PWM/PFM DS6121_DigOutType8_8: 2ex_L/1
  Ro1_or_Be2_PWM_L/1(Out1) -> PWM/PFM DS6121_DigOutType8_10: 4ex_L/2
  Ro1_or_Be2_PWM_H/1(Out1) -> PWM/PFM DS6121_DigOutType8_4: 4ex_H/2
  [PWM_frq_Hz] -> PWM/PFM DS6121_DigOutType8_3: 4pr_H/1
  [PWM_frq_Hz] -> PWM/PFM DS6121_DigOutType8_2: 2ex_H/1
  [PWM_enable] -> PWM/PFM DS6121_DigOutType8_7: 2pr_L/3
  [PWM_enable] -> PWM/PFM DS6121_DigOutType8_10: 4ex_L/3
  PWMfreq/1 -> [PWM_frq_Hz]
  Ro1_or_Be2_PWM_H/2(Out2) -> PWM/PFM DS6121_DigOutType8_1: 2pr_H/2
  [PWM_frq_Hz] -> PWM/PFM DS6121_DigOutType8_1: 2pr_H/1
  [PWM_enable] -> PWM/PFM DS6121_DigOutType8_2: 2ex_H/3
  [PWM_enable] -> PWM/PFM DS6121_DigOutType8_8: 2ex_L/3
  2%/1 -> PWMcompPositiv/1(In1)
  2%1/1 -> PWMcompNegativ/1(In1)
  PWMcompPositiv/1(PWMplusPositiv) -> Demux/1
  PWMcompNegativ/1(PWMplusNegativ) -> Demux1/1
  SET_Break/1 -> DS6121_DIO_MultBitOutType8_11: Break/1
  SET_valveSC/1 -> DS6121_DIO_MultBitOutType8_6: valveSC/1

== system FFT4dSpace_1/PA_tools_RepoInfo1 ==
  Ground : Ground
  Terminator : Terminator
  wires:
  Ground/1 -> Terminator/1

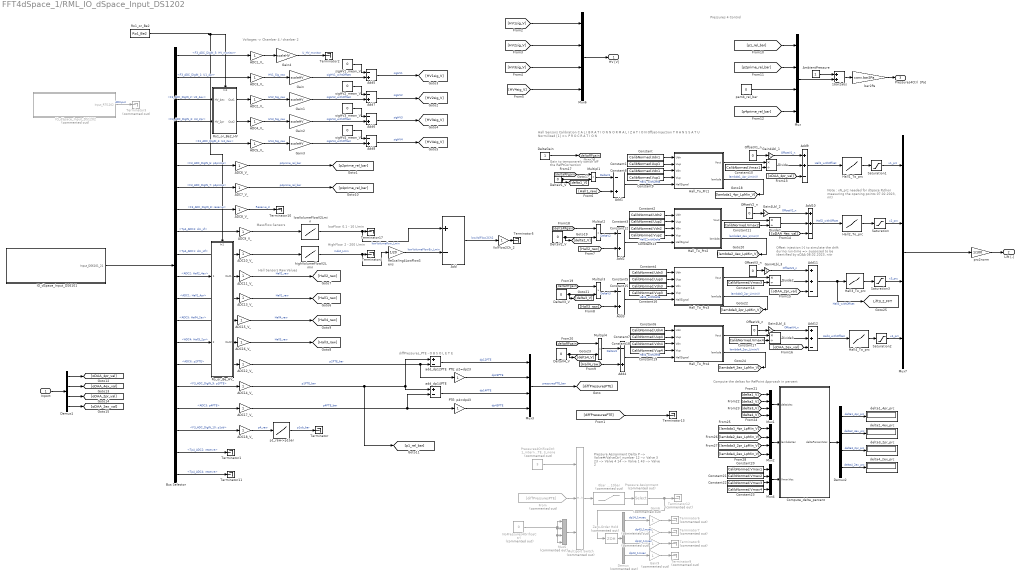
== system FFT4dSpace_1/RML_IO_dSpace_Input_DS1202 ==
  note: Compute the deltas for RefPoint Approach in percent
  note: Gain to temporarely switch off
      | the RefPtCorrection
  note: Offset injection [-] to simulate the drift
      | during run-time
      | => supposed to be identified by oDAA
      | 08.02.2023, nitr
  note: Note : xN_prz needed for dSpace Python
      | measuring the opening points
      | 07.02.2023, nitr
  note: Pressures 4 Control
  note: Hall Sensors Calibration                                                            C A L I B R A T I O N        N O R M A L I Z A T I O N    Offset-Injection               T R A N S              S A T U
      |                                                                                                                                                       Normilized [1]                                                   => P R O C         R A T I O N
  note: Hall Sensors Raw Values
  note: MassFlow Sensors
  note: HighFlow: 2 - 200 L/min
  note: diffPressures_PTE - O B S O L E T E
  note: lowFlow: 0.1 - 10 L/min
  note: Pressure Assignment
      |
      | Delta P --> Valve#/ValveCtrl_number
      | 12 --> Valve 3
      | 23 --> Valve 4
      | 14 --> Valve 1
      | 43 --> Valve 2
  note: Voltages -> Chamber 4 / chanber 2
  Inport : Inport
  "0bar ... 10bar " : Saturate  Commented=on  UpperLimit=10  LowerLimit=0
  1bar2abs : Sum
  ADC10_V_ : Gain
  ADC11_V_ : Gain
  ADC12_V_ : Gain
  ADC13_V_ : Gain
  ADC14_V_ : Gain
  ADC15_V_ : Gain
  ADC16_V_ : Gain
  ADC17_V_ : Gain
  ADC18_V_ : Gain
  ADC1_V_ : Gain
  ADC2_V_ : Gain
  ADC3_V_ : Gain
  ADC4_V_ : Gain
  ADC5_V_ : Gain
  ADC6_V_ : Gain
  ADC7_V_ : Gain
  ADC8_V_ : Gain
  ADC9_V_ : Gain
  Add : Sum  Inputs=+-
  Add{1..8} (8 alike) : Sum  Inputs=-+
  Add{9..12} (4 alike) : Sum  Inputs=++-
  AmbientPressure : Constant
  Bus Selector : BusSelector  OutputSignals=ADC_DIGin_DS6101_FLexIN_Type3.F3_ADC_DigIN_5: HV_monitor,ADC_DIGin_DS6101_FLexIN_Type3.F3_ADC_DigIN_1: U1_4pr,ADC_DIGin_DS6101_FLexIN_Type3.F3_ADC_DigIN_2: U2_4ex,ADC_DIGin_DS6101_FLexIN_Type3.F3_ADC_DigIN_3: U3_2pr,ADC_DIGin_DS6101_FLexIN_Type3.F3_ADC_DigIN_4: U4_2ex,ADC_DIGin_DS6101_FLexIN_Type3.F3_ADC_DigIN_6: p2prime,ADC_DIGin_DS6101_FLexIN_Type3.F3_ADC_DigIN_7: p4prime,ADC_DIGin_DS6101_FLexIN_Type3.F3_ADC_DigIN_8: reserve,ADC_DS6101_Type4.Tp4_ADC3: dm_Lf,ADC_DS6101_Type4.Tp4_ADC1: dm_Hf,ADC_DS6121_Type16.ADC2: Hall2_4ex,ADC_DS6121_Type16.ADC1: Hall1_4pr,ADC_DS6121_Type16.ADC5: Hall4_2ex,ADC_DS6121_Type16.ADC4: Hall3_2pr,ADC_DS6121_Type16.ADC6: p2PTE,ADC_DIGin_DS6101_FLexIN_Type3.F3_ADC_DigIN_9: p1PTE,ADC_DS6121_Type16.ADC3: p4PTE,ADC_DIGin_DS6101_FLexIN_Type3.F3_ADC_DigIN_10: p1ob,ADC_DS6101_Type4.Tp4_ADC2: reserve,ADC_DS6101_Type4.Tp4_ADC4: reserve
  Compute_delta_percent : MATLAB Function  TreatAsAtomicUnit=on
  Constant : Constant  Value=CalibNormed.Udn1
  Constant1 : Constant  Value=CalibNormed.Uup1
  Constant10 : Constant  Value=CalibNormed.Vmax1
  Constant11 : Constant  Value=CalibNormed.Vmax2
  Constant12 : Constant  Value=CalibNormed.Vdn2
  Constant13 : Constant  Value=CalibNormed.Vup2
  Constant14 : Constant  Value=CalibNormed.Vmax3
  Constant15 : Constant  Value=CalibNormed.Vdn3
  Constant16 : Constant  Value=CalibNormed.Vup3
  Constant17 : Constant  Value=CalibNormed.Vmax4
  Constant18 : Constant  Value=CalibNormed.Vdn4
  Constant19 : Constant  Value=CalibNormed.Vup4
  Constant2 : Constant  Value=CalibNormed.Udn2
  Constant20 : Constant  Value=CalibNormed.Vmax1
  Constant21 : Constant  Value=CalibNormed.Vmax2
  Constant22 : Constant  Value=CalibNormed.Vmax3
  Constant23 : Constant  Value=CalibNormed.Vmax4
  Constant3 : Constant  Value=CalibNormed.Uup2
  Constant4 : Constant  Value=CalibNormed.Udn3
  Constant5 : Constant  Value=CalibNormed.Uup3
  Constant6 : Constant  Value=CalibNormed.Udn4
  Constant7 : Constant  Value=CalibNormed.Uup4
  Constant8 : Constant  Value=CalibNormed.Vdn1
  Constant9 : Constant  Value=CalibNormed.Vup1
  DeltaGain : Constant
  DeltaV1_V : Constant  Value=0
  DeltaV2_V : Constant  Value=0
  DeltaV3_V : Constant  Value=0
  DeltaV4_V : Constant  Value=0
  Demux : Demux  Commented=on
  Demux1 : Demux
  Demux2 : Demux
  Divide{,1..3} (4 alike) : Product  Inputs=*/
  From : From  Commented=on  GotoTag=diffPressuresPTE
  Gain{,1..4} (5 alike) : Gain  Gain=scaleHV
  Gain4Lbl_{1..4} (4 alike) : Gain
  Gain{6..9} (4 alike) : Gain  Commented=on
  Hall1_To_prc : Lookup_n-D  NumberOfTableDimensions=1  BreakpointsForDimension1=[0 1]  Table=[0 100]  InternalRulePriority=Speed  RndMeth=Simplest  InputSameDT=on
  Hall2_To_prc : Lookup_n-D  NumberOfTableDimensions=1  BreakpointsForDimension1=[0 1]  Table=[0 100]  InternalRulePriority=Speed  RndMeth=Simplest  InputSameDT=on
  Hall3_To_prc : Lookup_n-D  NumberOfTableDimensions=1  BreakpointsForDimension1=[0 1]  Table=[0 100]  InternalRulePriority=Speed  RndMeth=Simplest  InputSameDT=on
  Hall4_To_prc : Lookup_n-D  NumberOfTableDimensions=1  BreakpointsForDimension1=[0 1]  Table=[0 100]  InternalRulePriority=Speed  RndMeth=Simplest  InputSameDT=on
  Hall_To_Prc1 : MATLAB Function  TreatAsAtomicUnit=on
  Hall_To_Prc2 : MATLAB Function  TreatAsAtomicUnit=on
  Hall_To_Prc3 : MATLAB Function  TreatAsAtomicUnit=on
  Hall_To_Prc4 : MATLAB Function  TreatAsAtomicUnit=on
  IO_dSpace_Input_DS1202 : Subsystem  Tag=PA_IO_dSpace_Input_DS1513  Commented=on  mask(PA_dSpace_Input_DS1513){}
      mask help:
      | This block contains all inputsignals from dSpace RTI 1401
      |
      | The signal types are:
      |
      | DIG_IN1 ... DIG_IN7
      | ADC1 ... ADC16
      | PWM9 ... PWM15
      |
      | The signals are muxed on a bus.
      mask Help: eval(['run(strcat(''',getenv('Festo2dSpace'),''',''\documentation\HelpForF2dSpaceElements.m''))']);
      mask Display: image('dSpaceInOut_rti1202_in.png')
  IO_dSpace_Input_DS6101 : Subsystem
      mask Display:
      | % image('dSpaceInOut_rti1202_in.png')
      | image('dSpace_input.png')
  Multipl{1..4} (4 alike) : Product  Inputs=**
  Multiport Switch : MultiPortSwitch  Commented=on  DataPortOrder=Specify indices  DataPortIndices={2,3}
  Mux{,1..4,6..7} (7 alike) : Mux
  Mux5 : Mux  Commented=on
  NoPressures4OrificeCtrl : Constant  Commented=on  Value=0
  OffsetV1_n : Constant  Value=0
  OffsetV2_n : Constant  Value=0
  OffsetV3_n : Constant  Value=0
  OffsetV4_n : Constant  Value=0
  PTE: p2=dp23 : Gain
  PTE: p4=dp43 : Gain
  Pressure Assignment : Selector  Commented=on  InputPortWidth=4  IndexOptions=Index vector (dialog)  Indices=[3 4 1 2]  OutputSizes=1
  "Pressures4OrificeCtrl: 1_intern, 2_PTE, 3_none" : Constant  Commented=on  Value=3
  ReScaling4LowFlowSens : Gain  Gain=1/20
  Ro1_or_Be2 : Constant  Value=Ro1_Be2
  Ro1_or_Be2_HV : Subsystem
      settings: PortSchema="{\"entries\":[{\"content\":{\"sides\":[{\"content\":{\"connectorIds\":[\"In1\",\"In2\"]},\"type\":\"ConnectorPlacement.EquallySpacedRectSide\",\"uuid\":\"33d120dc-88df-47e4-aceb-bf4939cbf745\"},{\"content\":{\"connectorIds\":[\"Out1\",\"Out2\"],\"side\":\"RIGHT\"},\"type\":\"ConnectorPlacement.EquallySpacedRectSide\",\"uuid\":\"b0000f29-fcf7-4c5a-a30f-88f0f10b005c\"},{\"content\":{\"connectorIds\":[\"In3\"],\"side\":\"TOP\"},\"type\":\"ConnectorPlacement.EquallySpacedRectSide\",\"uuid\":\"c9d41a43-30b6-47f1-b750-b85244b1e24d\"}]},\"type\":\"ConnectorPlacement.EquallySpacedConnector\",\"uuid\":\"b94f8a7b-aafd-4e61-9282-ebe0205f7a66\"}],\"packageUris\":[\"http://schema.mathworks.com/mf0/Connector/R2020b\"],\"version\":\"1.0\"}"
  Ro_or_Be_HV_ : Subsystem
      settings: PortSchema="{\"entries\":[{\"content\":{\"sides\":[{\"content\":{\"connectorIds\":[\"In1\",\"In2\"]},\"type\":\"ConnectorPlacement.EquallySpacedRectSide\",\"uuid\":\"33d120dc-88df-47e4-aceb-bf4939cbf745\"},{\"content\":{\"connectorIds\":[\"Out1\",\"Out2\"],\"side\":\"RIGHT\"},\"type\":\"ConnectorPlacement.EquallySpacedRectSide\",\"uuid\":\"b0000f29-fcf7-4c5a-a30f-88f0f10b005c\"},{\"content\":{\"connectorIds\":[\"In3\"],\"side\":\"TOP\"},\"type\":\"ConnectorPlacement.EquallySpacedRectSide\",\"uuid\":\"c9d41a43-30b6-47f1-b750-b85244b1e24d\"}]},\"type\":\"ConnectorPlacement.EquallySpacedConnector\",\"uuid\":\"b94f8a7b-aafd-4e61-9282-ebe0205f7a66\"}],\"packageUris\":[\"http://schema.mathworks.com/mf0/Connector/R2020b\"],\"version\":\"1.0\"}"
  Saturation{,1..3} (4 alike) : Saturate  UpperLimit=150  LowerLimit=-20
  Terminator{,1..2,4..5,10..11,13,17} (9 alike) : Terminator
  Terminator{3,6..9,12} (6 alike) : Terminator  Commented=on
  VolFlow2Ch_2 : Gain
  Zero-Order Hold : ZeroOrderHold  Commented=on  SampleTime=1e-3
  add_dp12PTE : Sum  Inputs=+-
  add_dp14PTE : Sum  Inputs=+-
  bar2Pa : Gain  Gain=conv.bar2Pa
  delta1_4pr_prc : Display
  delta2_4ex_prc : Display
  delta3_2pr_prc : Display
  delta4_2ex_prc : Display
  highVolumeFlowV2Lmin : Lookup_n-D  NumberOfTableDimensions=1  BreakpointsForDimension1=[0 10]  Table=[0 200]  InternalRulePriority=Speed  RndMeth=Simplest  InputSameDT=on
  lowVolumeFlowV2Lmin : Lookup_n-D  NumberOfTableDimensions=1  BreakpointsForDimension1=[0 10]  Table=[0 10]  InternalRulePriority=Speed  RndMeth=Simplest  InputSameDT=on
  p1_raw->p1bar : Lookup_n-D  NumberOfTableDimensions=1  BreakpointsForDimension1=[0.3 3]  Table=[0 7]  InternalRulePriority=Speed  RndMeth=Simplest  InputSameDT=on
  pamb_rel_bar : Constant  Value=0
  prz2norm : Gain  Gain=1/100
  sigHV1_mean_V : Constant  Value=0
  sigHV2_mean_V : Constant  Value=0
  sigHV3_mean_V : Constant  Value=0
  sigHV4_mean_V : Constant  Value=0
  HV [V] : Outport  VectorParamsAs1DForOutWhenUnconnected=off
  Lift [-] : Outport  Port=2  VectorParamsAs1DForOutWhenUnconnected=off
  Pressures4Ctrl  [Pa] : Outport  Port=3  VectorParamsAs1DForOutWhenUnconnected=off
  tag scope: Lift3_2_FFT=global
  wires:
  ADC14_V_/1 -> [p1_rel_bar], add_dp12PTE/1, add_dp14PTE/1  "p1PTE_bar"
  ADC2_V_/1 -> Gain1/1  "HV2_Sig_raw"
  ADC18_V_/1 -> p1_raw->p1bar/1  "p4_raw"
  Hall2_To_prc/1 -> Saturation/1
  Hall1_To_prc/1 -> Saturation1/1
  ADC17_V_/1 -> add_dp14PTE/2, PTE: p4=dp43/1  "p4PTE_bar"
  ADC12_V_/1 -> PTE: p2=dp23/1, add_dp12PTE/2  "p2PTE_bar"
  ADC4_V_/1 -> Gain2/1  "HV3_Sig_raw"
  lowVolumeFlowV2Lmin/1 -> Add/1, Terminator17/1  "lowVolumeflow_Lmin"
  ADC3_V_/1 -> Gain/1  "HV1_Sig_raw"
  ADC5_V_/1 -> Gain3/1  "HV4_Sig_raw"
  Hall4_To_prc/1 -> Saturation2/1
  Multiport Switch/1 -> "0bar ... 10bar "/1
  add_dp12PTE/1 -> Mux3/1  "dp12PTE"
  NoPressures4OrificeCtrl/1 -> Mux5/4, Mux5/3, Mux5/2, Mux5/1
  "Pressures4OrificeCtrl: 1_intern, 2_PTE, 3_none"/1 -> Multiport Switch/1
  add_dp14PTE/1 -> Mux3/3  "dp14PTE"
  Mux5/1 -> Multiport Switch/3
  bar2Pa/1 -> Pressures4Ctrl  [Pa]/1
  PTE: p2=dp23/1 -> Mux3/2  "dp23PTE"
  PTE: p4=dp43/1 -> Mux3/4  "dp43PTE"
  Mux3/1 -> [diffPressuresPTE]  "pressuresPTE_bar"
  Mux6/1 -> HV [V]/1
  highVolumeFlowV2Lmin/1 -> ReScaling4LowFlowSens/1, Terminator4/1  "mdot_Lmin"
  ADC1_V_/1 -> Gain4/1
  Gain4/1 -> Terminator2/1  "U_HV_monitor"
  "0bar ... 10bar "/1 -> Pressure Assignment/1
  Zero-Order Hold/1 -> Demux/1
  Demux/1 -> Gain6/1  "dp14_1msec"
  Demux/2 -> Gain7/1  "dp43_1msec"
  Demux/3 -> Gain8/1  "dp12_1msec"
  Demux/4 -> Gain9/1  "dp23_1msec"
  Gain6/1 -> Terminator6/1
  Gain7/1 -> Terminator7/1
  Gain8/1 -> Terminator8/1
  Gain9/1 -> Terminator9/1
  From/1 -> Multiport Switch/2
  Bus Selector/9 -> ADC9_V_/1  "<Tp4_ADC3: dm_Lf>"
  Bus Selector/16 -> ADC14_V_/1  "<F3_ADC_DigIN_9: p1PTE>"
  Bus Selector/10 -> ADC10_V_/1  "<Tp4_ADC1: dm_Hf>"
  Bus Selector/17 -> ADC17_V_/1  "<ADC3: p4PTE>"
  ADC9_V_/1 -> lowVolumeFlowV2Lmin/1
  ADC10_V_/1 -> highVolumeFlowV2Lmin/1
  Bus Selector/15 -> ADC12_V_/1  "<ADC6: p2PTE>"
  Bus Selector/1 -> ADC1_V_/1  "<F3_ADC_DigIN_5: HV_monitor>"
  [HV1sig_V] -> Mux6/1
  [HV2sig_V] -> Mux6/2
  [HV3sig_V] -> Mux6/3
  [HV4sig_V] -> Mux6/4
  Bus Selector/18 -> ADC18_V_/1  "<F3_ADC_DigIN_10: p1ob>"
  Bus Selector/2 -> ADC3_V_/1  "<F3_ADC_DigIN_1: U1_4pr>"
  Bus Selector/5 -> ADC5_V_/1  "<F3_ADC_DigIN_4: U4_2ex>"
  p1_raw->p1bar/1 -> Terminator/1  "p1ob_bar"
  Bus Selector/6 -> ADC6_V_/1  "<F3_ADC_DigIN_6: p2prime>"
  ADC6_V_/1 -> [p2prime_rel_bar]  "p2prime_rel_bar"
  ADC7_V_/1 -> [p4prime_rel_bar]  "p4prime_rel_bar"
  Bus Selector/7 -> ADC7_V_/1  "<F3_ADC_DigIN_7: p4prime>"
  Bus Selector/8 -> ADC8_V_/1  "<F3_ADC_DigIN_8: reserve>"
  ADC8_V_/1 -> Terminator10/1  "Reserve_3"
  Bus Selector/14 -> Ro_or_Be_HV_/2(Hall_2pr)  "<ADC4: Hall3_2pr>"
  Bus Selector/13 -> ADC15_V_/1  "<ADC5: Hall4_2ex>"
  Bus Selector/11 -> Ro_or_Be_HV_/1(Hall_4ex)  "<ADC2: Hall2_4ex>"
  Bus Selector/12 -> ADC13_V_/1  "<ADC1: Hall1_4pr>"
  Saturation/1 -> Mux7/2  "x2_prz"
  ADC11_V_/1 -> [Hall2_raw]  "Hall2_raw"
  Saturation1/1 -> Mux7/1  "x1_prz"
  ADC13_V_/1 -> [Hall1_raw]  "Hall1_raw"
  Saturation2/1 -> Mux7/4  "x4_prz"
  ADC15_V_/1 -> [Hall4_raw]  "Hall4_raw"
  Saturation3/1 -> Mux7/3  "x3_prz"
  ADC16_V_/1 -> [Hall3_raw]  "Hall3_raw"
  Constant/1 -> Hall_To_Prc1/1(Udn)
  Constant1/1 -> Hall_To_Prc1/2(Uup)
  Hall_To_Prc1/1(Vout) -> Divide/1
  Constant2/1 -> Hall_To_Prc2/1(Udn)
  Constant3/1 -> Hall_To_Prc2/2(Uup)
  Add2/1 -> Hall_To_Prc2/5(HallSignal)  "Hall2_withDelta"
  Hall3_To_prc/1 -> Saturation3/1
  Add3/1 -> Hall_To_Prc3/5(HallSignal)  "Hall3_withDelta"
  Constant6/1 -> Hall_To_Prc4/1(Udn)
  Add4/1 -> Hall_To_Prc4/5(HallSignal)  "Hall4_withDelta"
  Ro1_or_Be2_HV/1(Out1) -> ADC2_V_/1
  Ro1_or_Be2_HV/2(Out2) -> ADC4_V_/1
  Ro1_or_Be2/1 -> Ro1_or_Be2_HV/3(In1), Ro_or_Be_HV_/3(In1)
  Ro_or_Be_HV_/1(Out1) -> ADC11_V_/1
  Ro_or_Be_HV_/2(Out2) -> ADC16_V_/1
  Bus Selector/3 -> Ro1_or_Be2_HV/1(HV_4ex)  "<F3_ADC_DigIN_2: U2_4ex>"
  Bus Selector/4 -> Ro1_or_Be2_HV/2(HV_2pr)  "<F3_ADC_DigIN_3: U3_2pr>"
  IO_dSpace_Input_DS1202/1(Input_RTI1202) -> Terminator3/1  "ADInput"
  IO_dSpace_Input_DS6101/1(Input_DS6101_21) -> Bus Selector/1
  Bus Selector/19 -> Terminator1/1  "<Tp4_ADC2: reserve>"
  Bus Selector/20 -> Terminator11/1  "<Tp4_ADC4: reserve>"
  sigHV4_mean_V/1 -> Add8/1
  Add7/1 -> [HV2sig_V]  "sigHV2"
  sigHV1_mean_V/1 -> Add5/1
  sigHV3_mean_V/1 -> Add6/1
  sigHV2_mean_V/1 -> Add7/1
  Add6/1 -> [HV3sig_V]  "sigHV3"
  Add5/1 -> [HV1sig_V]  "sigHV1"
  Gain1/1 -> Add7/2  "sigHV2_withOffset"
  Gain/1 -> Add5/2  "sigHV1_wihtOffset"
  Gain3/1 -> Add8/2  "sigHV4_withOffset"
  Add8/1 -> [HV4sig_V]  "sigHV4"
  Gain2/1 -> Add6/2  "sigHV3_withOffset"
  [Hall1_raw] -> Add1/2
  [Hall4_raw] -> Add4/2
  [Hall3_raw] -> Add3/2
  [Hall2_raw] -> Add2/2
  Add1/1 -> Hall_To_Prc1/5(HallSignal)  "Hall1_withDelta"
  Constant8/1 -> Hall_To_Prc1/3(Vdn)
  Constant9/1 -> Hall_To_Prc1/4(Vup)
  Constant10/1 -> Divide/2
  Hall_To_Prc2/1(Vout) -> Divide1/1
  Constant12/1 -> Hall_To_Prc2/3(Vdn)
  Constant13/1 -> Hall_To_Prc2/4(Vup)
  Constant11/1 -> Divide1/2
  Hall_To_Prc3/1(Vout) -> Divide2/1
  Constant14/1 -> Divide2/2
  Constant4/1 -> Hall_To_Prc3/1(Udn)
  Constant5/1 -> Hall_To_Prc3/2(Uup)
  Constant15/1 -> Hall_To_Prc3/3(Vdn)
  Constant16/1 -> Hall_To_Prc3/4(Vup)
  Constant17/1 -> Divide3/2
  Hall_To_Prc4/1(Vout) -> Divide3/1
  Constant7/1 -> Hall_To_Prc4/2(Uup)
  Constant18/1 -> Hall_To_Prc4/3(Vdn)
  Constant19/1 -> Hall_To_Prc4/4(Vup)
  Pressure Assignment/1 -> Zero-Order Hold/1, Terminator12/1
  [diffPressuresPTE] -> Terminator13/1
  [p1_rel_bar] -> Mux/1
  [p2prime_rel_bar] -> Mux/2
  prz2norm/1 -> Lift [-]/1
  Mux7/1 -> prz2norm/1
  Divide/1 -> Add9/2
  Add9/1 -> Hall1_To_prc/1  "Hall1_withOffset"
  Divide1/1 -> Add10/2
  OffsetV2_n/1 -> Gain4Lbl_2/1
  Add10/1 -> Hall2_To_prc/1  "Hall2_withOffset"
  Divide2/1 -> Add11/2
  Add11/1 -> [Lift3_2_FFT], Hall3_To_prc/1  "Hall3_withOffset"
  Divide3/1 -> Add12/2
  OffsetV4_n/1 -> Gain4Lbl_4/1
  Add12/1 -> Hall4_To_prc/1  "Hall4_withOffset"
  1bar2abs/1 -> bar2Pa/1
  Mux/1 -> 1bar2abs/2
  AmbientPressure/1 -> 1bar2abs/1
  [p4prime_rel_bar] -> Mux/4
  pamb_rel_bar/1 -> Mux/3
  Demux1/2 -> [oDAA_4ex_val]
  Demux1/1 -> [oDAA_4pr_val]
  Demux1/4 -> [oDAA_2ex_val]
  Inport/1 -> Demux1/1
  Demux1/3 -> [oDAA_2pr_val]
  [oDAA_4pr_val] -> Add9/3
  [oDAA_4ex_val] -> Add10/3
  [oDAA_2pr_val] -> Add11/3
  [oDAA_2ex_val] -> Add12/3
  Gain4Lbl_1/1 -> Add9/1  "OffsetV1_n"
  OffsetV1_n/1 -> Gain4Lbl_1/1
  Gain4Lbl_2/1 -> Add10/1  "OffsetV2_n"
  OffsetV3_n/1 -> Gain4Lbl_3/1
  Gain4Lbl_3/1 -> Add11/1  "OffsetV3_n"
  Gain4Lbl_4/1 -> Add12/1  "OffsetV4_n"
  DeltaV1_V/1 -> [delta1_V], Multipl1/2
  Multipl1/1 -> Add1/1  "DeltaV1"
  DeltaGain/1 -> [deltaRFgain]
  [deltaRFgain] -> Multipl1/1
  Multipl2/1 -> Add2/1  "DeltaV2"
  DeltaV2_V/1 -> [delta2_V], Multipl2/2
  [deltaRFgain] -> Multipl2/1
  [deltaRFgain] -> Multipl3/1
  Multipl3/1 -> Add3/1  "DeltaV3"
  DeltaV3_V/1 -> [delta3_V], Multipl3/2
  [deltaRFgain] -> Multipl4/1
  Multipl4/1 -> Add4/1  "DeltaV4"
  DeltaV4_V/1 -> [delta4_V], Multipl4/2
  Hall_To_Prc1/2(lambda) -> [lambda1_4pr_LpMin_V]  "lambda1_4pr_L/min/V"
  Hall_To_Prc2/2(lambda) -> [lambda2_4ex_LpMin_V]  "lambda2_4ex_L/min/V"
  Hall_To_Prc3/2(lambda) -> [lambda3_2pr_LpMin_V]  "lambda3_2pr_L/min/V"
  Hall_To_Prc4/2(lambda) -> [lambda4_2ex_LpMin_V]  "lambda4_2ex_L/min/V"
  [delta1_V] -> Mux1/1
  [delta2_V] -> Mux1/2
  [delta3_V] -> Mux1/3
  [delta4_V] -> Mux1/4
  [lambda1_4pr_LpMin_V] -> Mux2/1
  [lambda2_4ex_LpMin_V] -> Mux2/2
  [lambda3_2pr_LpMin_V] -> Mux2/3
  [lambda4_2ex_LpMin_V] -> Mux2/4
  Constant20/1 -> Mux4/1
  Constant21/1 -> Mux4/2
  Constant22/1 -> Mux4/3
  Constant23/1 -> Mux4/4
  Mux1/1 -> Compute_delta_percent/1(deltaVec)
  Mux2/1 -> Compute_delta_percent/2(lambdaVec)
  Mux4/1 -> Compute_delta_percent/3(VmaxVec)
  Compute_delta_percent/1(deltaPercentVec) -> Demux2/1
  Demux2/1 -> delta1_4pr_prc/1  "delta1_4pr_prc"
  Demux2/2 -> delta2_4ex_prc/1  "delta2_4ex_prc"
  Demux2/4 -> delta4_2ex_prc/1  "delta4_2ex_prc"
  Demux2/3 -> delta3_2pr_prc/1  "delta3_2pr_prc"
  ReScaling4LowFlowSens/1 -> Add/2  "lowVolumeFlowEx_Lmin"
  Add/1 -> VolFlow2Ch_2/1  "lowVolFlow2Ch2"
  VolFlow2Ch_2/1 -> Terminator5/1

== system FFT4dSpace_1/RML_tools_RepoInfo ==
  Ground : Ground
  Terminator : Terminator
  wires:
  Ground/1 -> Terminator/1
